simulink model "inverter"  (R2016b)
settings: Solver=VariableStepAuto  StartTime=0.0  StopTime=0.1  RelTol=1e-3
libraries: powerlib x11, powerlib_meascontrol x2, dspstat3 x2, simulink x1
settings Model: Creator=lenovo  LastModifiedBy=lenovo

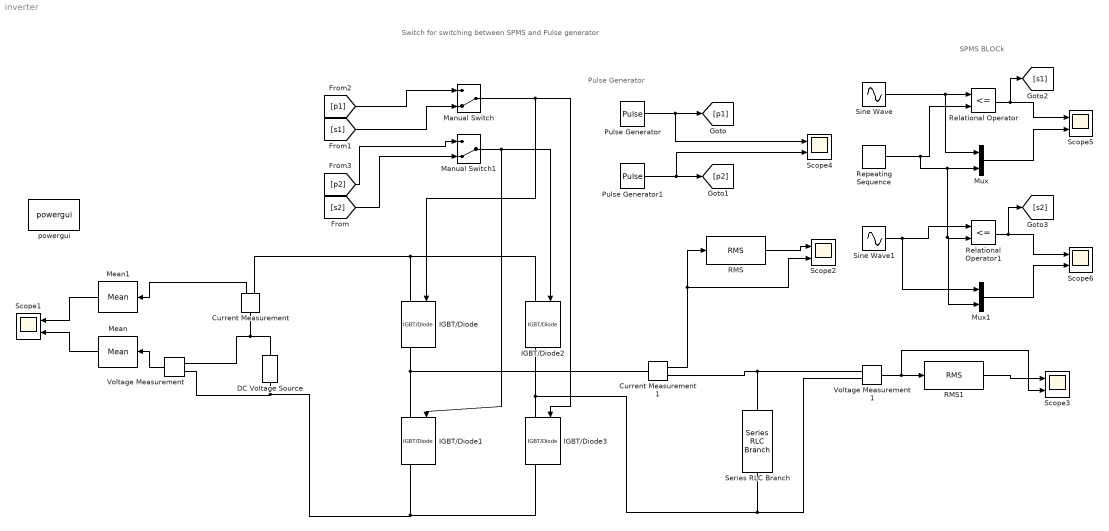
== system inverter ==
  note: Switch for switching between SPMS and Pulse generator
  note: Pulse Generator
  note: SPMS BLOCk
  Current Measurement : powerlib/Measurements/Current Measurement  PhasorSimulation=off  OutputType=Complex  PSBequivalent=0
  Current Measurement1 : powerlib/Measurements/Current Measurement  PhasorSimulation=off  OutputType=Complex  PSBequivalent=0
  DC Voltage Source : powerlib/Electrical Sources/DC Voltage Source  Amplitude=100  Measurements=None
  IGBT/Diode{,1..3} (4 alike) : powerlib/Power Electronics/IGBT//Diode  Ron=1e-3  Rs=1e5  Cs=inf  Measurements=on
  Manual Switch : ManualSwitch  CurrentSetting=0
  Manual Switch1 : ManualSwitch  CurrentSetting=0
  Mean : powerlib_meascontrol/Measurements/Mean  Freq=60  Vinit=0  Ts=0
  Mean1 : powerlib_meascontrol/Measurements/Mean  Freq=60  Vinit=0  Ts=0
  Mux : Mux  Inputs=2
  Mux1 : Mux  Inputs=2
  Pulse Generator : DiscretePulseGenerator  PulseType=Time based  Period=1/50  PulseWidth=50
  Pulse Generator1 : DiscretePulseGenerator  PulseType=Time based  Period=1/50  PulseWidth=50  PhaseDelay=0.01
  RMS : dspstat3/RMS  run=off  directionMode=Each column  dimension=1  InputProcessing=Columns as channels (frame based)  reset_popup=None
  RMS1 : dspstat3/RMS  run=off  directionMode=Each column  dimension=1  InputProcessing=Columns as channels (frame based)  reset_popup=None
  Relational Operator : RelationalOperator  Operator=<=  OutDataTypeStr=boolean  RndMeth=Simplest
  Relational Operator1 : RelationalOperator  Operator=<=  OutDataTypeStr=boolean  RndMeth=Simplest
  Repeating Sequence : simulink/Sources/Repeating Sequence  rep_seq_t=[0 0.5/5000 1/5000]  rep_seq_y=[0 1 0]
  Scope{1..6} (6 alike) : Scope  NumInputPorts=2
  Series RLC Branch : powerlib/Elements/Series RLC Branch  LConnTagsString=__new0  RConnTagsString=__new0  BranchType=R  Resistance=50  Inductance=0.001  SetiL0=off  InitialCurrent=0  Capacitance=1e-6  Setx0=off  InitialVoltage=0  Measurements=None
  Sine Wave : Sin  Frequency=2*pi*50  SampleTime=50e-6
  Sine Wave1 : Sin  Amplitude=-1  Frequency=2*pi*50  SampleTime=50e-6
  Voltage Measurement : powerlib/Measurements/Voltage Measurement  PhasorSimulation=off  OutputType=Complex  PSBequivalent=0
  Voltage Measurement1 : powerlib/Measurements/Voltage Measurement  PhasorSimulation=off  OutputType=Complex  PSBequivalent=0
  powergui : powerlib/powergui  Priority=1  SimulationMode=Continuous  SolverType=Tustin/Backward Euler (TBE)  SampleTime=50e-6  frequency=60  SPID=off  DisableSnubberDevices=off  DisableRonSwitches=off  DisableVfSwitches=off  SwTol=0  DisplayEquations=off  Interpol=off  ExternalGateDelay=off  methode=off  Ts=10  FunctionMessages=off  echomessages=off  HookPort=off  EnableUseOfTLC=off  x0status=blocks  frequencyindice=0  Pbase=100e6  ErrMax=1e-4  Iterations=50  UnitsV=kV  UnitsW=MW  buscounter=0  RestoreLinks=warning  ResistiveCurrentMeasurement=off  Frange=[0:2:500]  Ylog=off  Xlog=on  ShowGrid=off  save=off  variable=ZData  structure=0  ZoomFFT=off  StartTime=0.0  cycles=1  DisplayStyle=1  fundamental=60  FreqAxis=off  MaxFrequency=1000  frequencyindicesteady=1  RmsSteady=1  display=off
  wires:
  Voltage Measurement/1 -> Mean/1
  Current Measurement/1 -> Mean1/1
  Current Measurement1/1 -> Scope2/2, RMS/1
  RMS/1 -> Scope2/1
  RMS1/1 -> Scope3/1
  Voltage Measurement1/1 -> Scope3/2, RMS1/1
  Pulse Generator/1 -> Scope4/1, [p1]
  Pulse Generator1/1 -> Scope4/2, [p2]
  Mean1/1 -> Scope1/1
  Mean/1 -> Scope1/2
  Sine Wave/1 -> Mux/1, Relational Operator/1
  Relational Operator/1 -> [s1], Scope5/1
  Mux/1 -> Scope5/2
  Relational Operator1/1 -> [s2], Scope6/1
  Mux1/1 -> Scope6/2
  Sine Wave1/1 -> Mux1/1, Relational Operator1/1
  Repeating Sequence/1 -> Mux1/2, Relational Operator1/2, Mux/2, Relational Operator/2
  [p1] -> Manual Switch/1
  [p2] -> Manual Switch1/1
  [s1] -> Manual Switch/2
  Manual Switch/1 -> IGBT/Diode/1, IGBT/Diode3/1
  [s2] -> Manual Switch1/2
  Manual Switch1/1 -> IGBT/Diode1/1, IGBT/Diode2/1
  connections:
  Voltage Measurement/LConn2 -- Current Measurement/LConn1 -- DC Voltage Source/RConn1
  DC Voltage Source/LConn1 -- IGBT/Diode3/RConn1 -- IGBT/Diode1/RConn1 -- Voltage Measurement/LConn1
  Current Measurement/RConn1 -- IGBT/Diode/LConn1 -- IGBT/Diode2/LConn1
  IGBT/Diode/RConn1 -- Current Measurement1/LConn1 -- IGBT/Diode1/LConn1
  IGBT/Diode2/RConn1 -- Series RLC Branch/RConn1 -- Voltage Measurement1/LConn2 -- IGBT/Diode3/LConn1
  Current Measurement1/RConn1 -- Series RLC Branch/LConn1 -- Voltage Measurement1/LConn1
